simulink model "GalvoModel_v3_discret_simo"  (R2013a)
settings: Solver=ode45  StartTime=0.0  StopTime=20e-3  RelTol=1e-3
PreLoadFcn:
  | RIN=evalin('base',param.RIN);
  | TRC=evalin('base',param.TRC);
  | CR=evalin('base',param.CR);
  | CL=evalin('base',param.CL);
  | FR=evalin('base',param.FR);
  | KTR=evalin('base',param.KTR);
  | BEM=evalin('base',param.BEM);
InitFcn:
  | RIN=evalin('base',param.RIN);
  | TRC=evalin('base',param.TRC);
  | CR=evalin('base',param.CR);
  | CL=evalin('base',param.CL);
  | FR=evalin('base',param.FR);
  | KTR=evalin('base',param.KTR);
  | BEM=evalin('base',param.BEM);
model workspace (MAT data in the model file):
  Var = 0
values from neighbouring files (symbols this model uses):
  param = loadGalvoParam(4)    [Compare_multiphys_blockdiag.m]    (also in DcMotorPosition_v1.m = {; GalvoModel_WOK_step.m = {; GalvoModel_v31_reference_procs.m = loadGalvoParam([]); GalvoModel_v3_discret_proc.m = {)
libraries: simulink x2
settings Model: BufferReuse=off  Creator=mainster  LastModifiedBy=mainster
settings OptimizationCC: InlineParams=on  BufferReuse=off
settings DebuggingCC: SolverPrmCheckMsg=none  InitInArrayFormatMsg=none

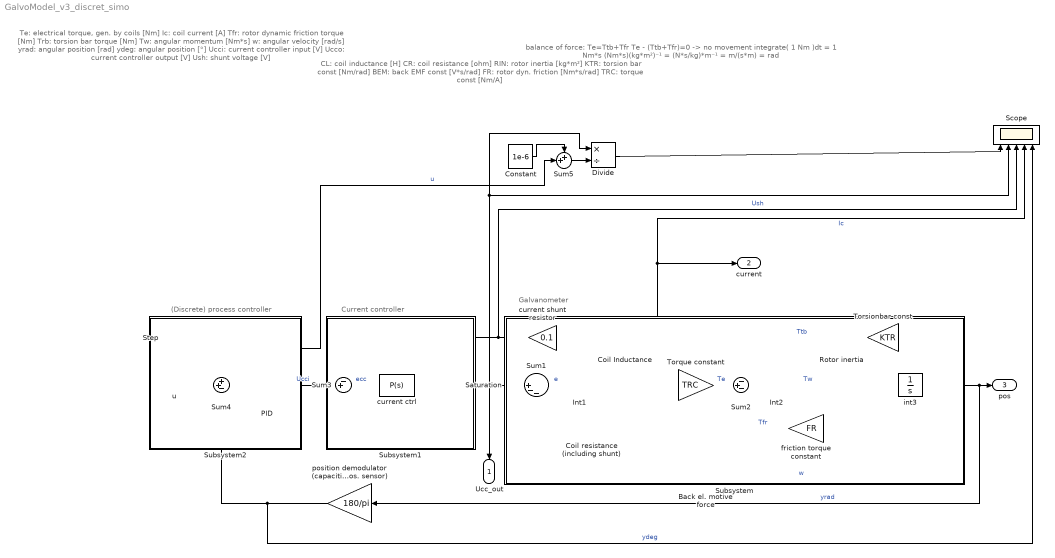
== system GalvoModel_v3_discret_simo ==
  note: Current controller
  note: Galvanometer
  note: Te: 		electrical torque, gen. by coils		[Nm]
      |  Ic: 			coil current							[A]
      |  Tfr:		rotor dynamic friction torque 		[Nm]
      |  Trb:		torsion bar torque					[Nm]
      |  Tw:		angular momentum				[Nm*s]
      |  w:			angular velocity 					[rad/s]
      |  yrad:		angular position 					[rad]
      |  ydeg:		angular position 					[°]
      |  Ucci:		current controller input				[V]
      |  Ucco:		current controller output			[V]
      |  Ush:		shunt voltage						[V]
  note: CL:	coil inductance 		[H]
      |  CR:	coil resistance 			[ohm]
      |  RIN:	rotor inertia 			[kg*m²]
      |  KTR:	torsion bar const 		[Nm/rad]
      |  BEM:	back EMF const		[V*s/rad]
      |  FR:	rotor dyn. friction		[Nm*s/rad]
      |  TRC:	torque const			[Nm/A]
  note: balance of force: 	Te=Ttb+Tfr
      | 					Te - (Ttb+Tfr)=0  ->  no movement
      |
      |  integrate( 1 Nm )dt = 1 Nm*s
      |  (Nm*s)(kg*m²)⁻¹ = (N*s/kg)*m⁻¹ = m/(s*m) = rad
  note: (Discrete) process controller
  u : Inport
  Back el. motive force : Gain  Gain=BEM
  Coil Inductance : Gain  Gain=1/CL
  Coil resistance (including shunt) : Gain  Gain=CR
  Constant : Constant  Value=1e-6
  Divide : Product  Inputs=*/
  Int1 : Integrator
  Int2 : Integrator
  PID : simulink/Continuous/PID Controller  Controller=PID  TimeDomain=Continuous-time  SampleTime=1  IntegratorMethod=Forward Euler  FilterMethod=Forward Euler  Form=Parallel  P=0.118803398901385  I=41.4515194383798  D=8.41592067923308e-05  N=758717.459878032  InitialConditionSource=internal  InitialConditionForIntegrator=0  InitialConditionForFilter=0  ExternalReset=none  LimitOutput=on  UpperSaturationLimit=2.5  LowerSaturationLimit=-2.5  LinearizeAsGain=off  AntiWindupMode=none  Kb=1  TrackingMode=off  Kt=0  PParamMin=[]  PParamMax=[]  IParamMin=[]  IParamMax=[]  DParamMin=[]  DParamMax=[]  NParamMin=[]  NParamMax=[]  KbParamMin=[]  KbParamMax=[]  KtParamMin=[]  KtParamMax=[]  POutMin=[]  POutMax=[]  IOutMin=[]  IOutMax=[]  DOutMin=[]  DOutMax=[]  NOutMin=[]  NOutMax=[]  KbOutMin=[]  KbOutMax=[]  KtOutMin=[]  KtOutMax=[]  IntegratorOutMin=[]  IntegratorOutMax=[]  FilterOutMin=[]  FilterOutMax=[]  SumOutMin=[]  SumOutMax=[]  SumI1OutMin=[]  SumI1OutMax=[]  SumI2OutMin=[]  SumI2OutMax=[]  SumI3OutMin=[]  SumI3OutMax=[]  SumDOutMin=[]  SumDOutMax=[]  SaturationOutMin=[]  SaturationOutMax=[]  IntegratorContinuousStateAttributes=''  IntegratorStateMustResolveToSignalObject=off  IntegratorRTWStateStorageClass=Auto  FilterContinuousStateAttributes=''  FilterStateMustResolveToSignalObject=off  FilterRTWStateStorageClass=Auto
  Rotor inertia : Gain  Gain=1/RIN
  Saturation : Saturate  UpperLimit=25e0  LowerLimit=-25e0
      settings: AttributesFormatString=Saturation:\n<%<LowerLimit>\n>%<UpperLimit>
  Scope : Scope  NumInputPorts=5
      settings: ShowLegends=on  TimeRange=0.02  YMin=-30~-1~-0.2~-2~0  YMax=10~3~0.6~6~20  MaxDataPoints=500000
  Step : Step  Time=1e-3  After=20  SampleTime=0
      settings: AttributesFormatString=Ampl.: %<After>
  Subsystem : Subsystem  mask{d=0}
      mask Display: disp('')
  Subsystem1 : Subsystem  mask{d=0}
      mask Display: disp('')
  Subsystem2 : Subsystem  mask{d=0}
      mask Display: disp('')
  Sum1 : Sum  Inputs=||+--
  Sum2 : Sum  Inputs=-+-
  Sum3 : Sum  Inputs=-+|
  Sum4 : Sum  Inputs=++-
  Sum5 : Sum  Inputs=++|
  Torque constant : Gain  Gain=TRC
  Torsionbar const : Gain  Gain=KTR
  current ctrl : simulink/Continuous/PID Controller  Controller=P  TimeDomain=Continuous-time  SampleTime=1  IntegratorMethod=Forward Euler  FilterMethod=Forward Euler  Form=Parallel  P=10  I=0.7525  D=0.156  N=100  InitialConditionSource=internal  InitialConditionForIntegrator=0  InitialConditionForFilter=0  ExternalReset=none  LimitOutput=off  UpperSaturationLimit=25  LowerSaturationLimit=-25  LinearizeAsGain=off  AntiWindupMode=none  Kb=1  TrackingMode=off  Kt=1  PParamMin=[]  PParamMax=[]  IParamMin=[]  IParamMax=[]  DParamMin=[]  DParamMax=[]  NParamMin=[]  NParamMax=[]  KbParamMin=[]  KbParamMax=[]  KtParamMin=[]  KtParamMax=[]  POutMin=[]  POutMax=[]  IOutMin=[]  IOutMax=[]  DOutMin=[]  DOutMax=[]  NOutMin=[]  NOutMax=[]  KbOutMin=[]  KbOutMax=[]  KtOutMin=[]  KtOutMax=[]  IntegratorOutMin=[]  IntegratorOutMax=[]  FilterOutMin=[]  FilterOutMax=[]  SumOutMin=[]  SumOutMax=[]  SumI1OutMin=[]  SumI1OutMax=[]  SumI2OutMin=[]  SumI2OutMax=[]  SumI3OutMin=[]  SumI3OutMax=[]  SumDOutMin=[]  SumDOutMax=[]  SaturationOutMin=[]  SaturationOutMax=[]  IntegratorContinuousStateAttributes=''  IntegratorStateMustResolveToSignalObject=off  IntegratorRTWStateStorageClass=Auto  FilterContinuousStateAttributes=''  FilterStateMustResolveToSignalObject=off  FilterRTWStateStorageClass=Auto
  current shunt resistor : Gain  Gain=0.1
  friction torque constant : Gain  Gain=FR
  int3 : Integrator
  position demodulator (capacitive angular pos. sensor) : Gain  Gain=180/pi
  Ucc_out : Outport
  current : Outport  Port=2
  pos : Outport  Port=3
  wires:
  int3/1 -> Torsionbar const/1, pos/1, position demodulator (capacitive angular pos. sensor)/1  "yrad"
  Torque constant/1 -> Sum2/2  "Te"
  Sum3/1 -> current ctrl/1  "ecc"
  current shunt resistor/1 -> Scope/3, Sum3/1  "Ush"
  PID/1 -> Sum3/2  "Ucci"
  Sum4/1 -> PID/1
  Coil Inductance/1 -> current/1, Scope/4, current shunt resistor/1, Coil resistance (including shunt)/1, Torque constant/1  "Ic"
  Torsionbar const/1 -> Sum2/1  "Ttb"
  current ctrl/1 -> Saturation/1
  Step/1 -> Sum4/1
  u/1 -> Sum5/2, Sum4/2  "u"
  position demodulator (capacitive angular pos. sensor)/1 -> Sum4/3, Scope/5  "ydeg"
  Int1/1 -> Coil Inductance/1
  Coil resistance (including shunt)/1 -> Sum1/3
  Sum1/1 -> Int1/1  "e"
  Int2/1 -> Rotor inertia/1  "Tw"
  Sum2/1 -> Int2/1
  Rotor inertia/1 -> int3/1, Back el. motive force/1, friction torque constant/1  "w"
  friction torque constant/1 -> Sum2/3  "Tfr"
  Back el. motive force/1 -> Sum1/2
  Saturation/1 -> Ucc_out/1, Divide/1, Scope/2, Sum1/1
  Divide/1 -> Scope/1
  Constant/1 -> Sum5/1
  Sum5/1 -> Divide/2

== system GalvoModel_v3_discret_simo/Subsystem ==

== system GalvoModel_v3_discret_simo/Subsystem1 ==

== system GalvoModel_v3_discret_simo/Subsystem2 ==
